simulink model "HelicPlantMRAC"  (R2023b)
settings: Solver=ode45  StartTime=0.0  StopTime=100  RelTol=1e-3  EnableMultiTasking=on
values from neighbouring files (symbols this model uses):
  am = -4.0    (= -4)    [int.m]
  bbar = -1    [int.m]
  bm = 4.0    (= 4)    [int.m]
  gammaphi = 0.1    [int.m]
  gammar = 0.0005    [int.m]
  gammax = 0.0005    [int.m]
  ke = 10    [int.m]
  khat0 = 0    [int.m]
  lhat0 = 0    [int.m]
  p = -1/(2*am)    (= 0.125)    [int.m]
  R = 0.15    [int.m]
  sigma2e = 0.0    (= 0)    [int.m]
  Tc = 0.1    [int.m]
  thetahat0 = 0    [int.m]
  wr = 0.25    [int.m]
libraries: simulink x1
settings Model: Creator=Abel  LastModifiedBy=Abel
settings SolverCC: AlgebraicLoopSolver=TrustRegion
settings DataIOCC: LimitDataPoints=on  SaveFormat=Array  SignalLoggingSaveFormat=ModelDataLogs  ReturnWorkspaceOutputs=off
settings OptimizationCC: InitFltsAndDblsToZero=on  LifeSpan=inf
settings DebuggingCC: SaveWithParameterizedLinksMsg=none  UnderspecifiedInitializationDetection=Classic  MergeDetectMultiDrivingBlocksExec=none  SignalResolutionControl=TryResolveAllWithWarning  SolverPrmCheckMsg=warning  MultiTaskDSMMsg=warning  MultiTaskCondExecSysMsg=none  FcnCallInpInsideContextMsg=warning  UnconnectedInputMsg=warning  UnconnectedOutputMsg=warning  UnconnectedLineMsg=warning  SFUnexpectedBacktrackingDiag=warning  SFNoUnconditionalDefaultTransitionDiag=warning  SFExecutionAtInitializationDiag=none  ArithmeticOperatorsInVariantConditions=warning
settings HardwareCC: ProdBitPerPointer=32  ProdBitPerSizeT=32  ProdBitPerPtrDiffT=32  ProdLargestAtomicFloat=None  ProdIntDivRoundTo=Undefined  ProdEndianess=Unspecified  ProdWordSize=32  ProdHWDeviceType=32-bit Generic
settings ModelReferenceCC: PropagateSignalLabelsOutOfModel=off
settings CodeAppCC: StateflowObjectComments=on
settings GRTTargetCC: TargetFcnLib=ansi_tfl_tmw.mat  TargetLangStandard=C89/C90 (ANSI)  CombineOutputUpdateFcns=off  GRTInterface=on
settings ConfigComp: CovMetricSettings=dw  CovSaveCumulativeToWorkspaceVar=on  CovSaveSingleToWorkspaceVar=on

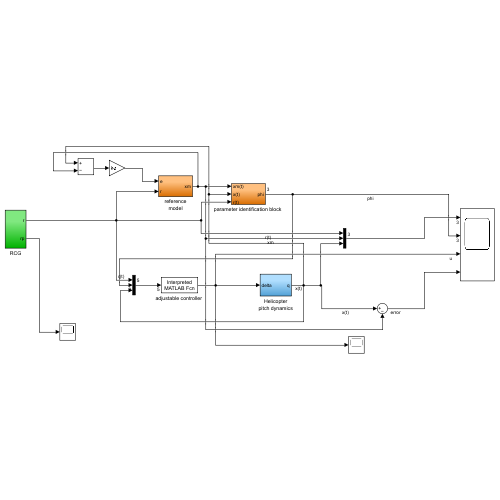
[thumbnail: Simulink's stored preview of the top-level diagram]
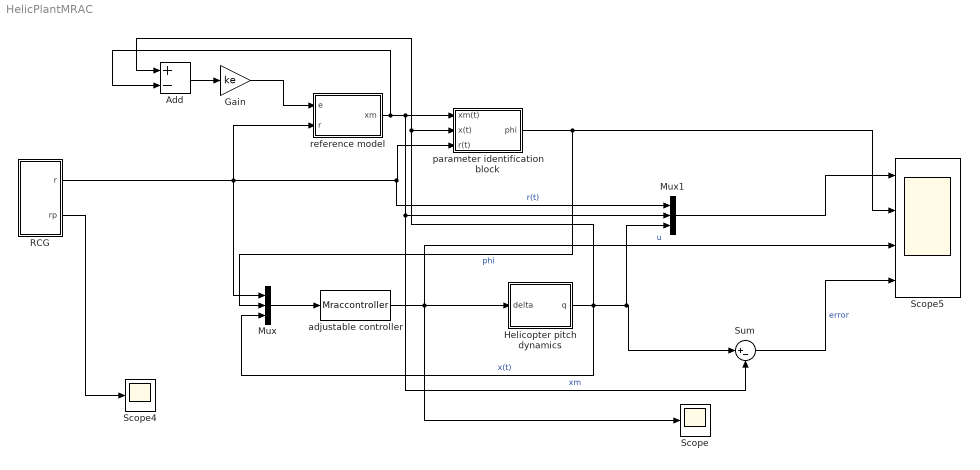
== system HelicPlantMRAC ==
  Add : Sum  Inputs=+-
  Gain : Gain  Gain=ke
  Helicopter pitch dynamics : Subsystem
  Mux : Mux  Inputs=[1 3 1]
  Mux1 : Mux  Inputs=3
  RCG : Subsystem
  Scope : Scope
  Scope4 : Scope
  Scope5 : Scope  NumInputPorts=4
  Sum : Sum  Inputs=|+-
  "adjustable controller " : MATLABFcn  MATLABFcn=Mraccontroller  OutputDimensions=1
  "parameter identification block " : Subsystem
  reference model : Subsystem
  wires:
  RCG/1(r) -> Mux/1, Mux1/1, "parameter identification block "/3(r(t)), reference model/2(r)  "r(t)"
  reference model/1(xm) -> Add/2, Sum/2, Mux1/2, "parameter identification block "/1(xm(t))  "xm"
  Helicopter pitch dynamics/1(q) -> Mux1/3, Sum/1, Mux/3, Add/1, "parameter identification block "/2(x(t))  "x(t)"
  "adjustable controller "/1 -> Scope5/3, Helicopter pitch dynamics/1(delta), Scope/1  "u"
  "parameter identification block "/1(phi) -> Scope5/2, Mux/2  "phi"
  Mux/1 -> "adjustable controller "/1
  RCG/2(rp) -> Scope4/1
  Add/1 -> Gain/1
  Gain/1 -> reference model/1(e)
  Mux1/1 -> Scope5/1
  Sum/1 -> Scope5/4  "error"

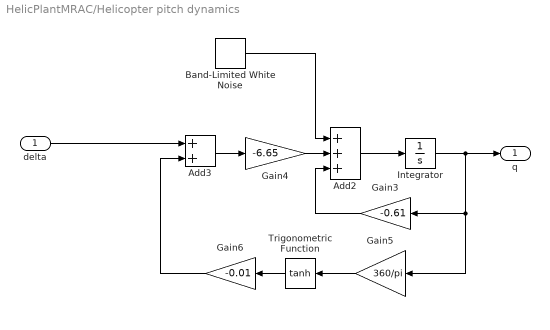
== system HelicPlantMRAC/Helicopter pitch dynamics ==
  delta : Inport
  Add2 : Sum  Inputs=+++
  Add3 : Sum
  Band-Limited White Noise : simulink/Sources/Band-Limited White Noise  Cov=[sigma2e*Tc]  Ts=Tc  seed=[23341]
  Gain3 : Gain  Gain=-0.61
  Gain4 : Gain  Gain=-6.65
  Gain5 : Gain  Gain=360/pi
  Gain6 : Gain  Gain=-0.01
  Integrator : Integrator
  Trigonometric Function : Trigonometry  Operator=tanh
  q : Outport
  wires:
  Integrator/1 -> Gain3/1, Gain5/1, q/1
  Add2/1 -> Integrator/1
  Gain5/1 -> Trigonometric Function/1
  Trigonometric Function/1 -> Gain6/1
  Add3/1 -> Gain4/1
  Gain6/1 -> Add3/2
  delta/1 -> Add3/1
  Gain3/1 -> Add2/3
  Gain4/1 -> Add2/2
  Band-Limited White Noise/1 -> Add2/1

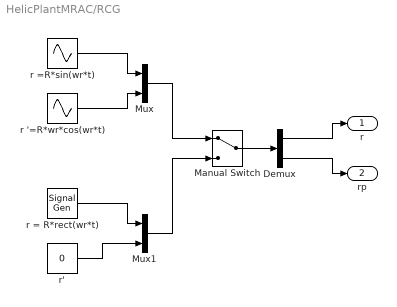
== system HelicPlantMRAC/RCG ==
  Demux : Demux  Outputs=2
  Manual Switch : ManualSwitch
  Mux : Mux  Inputs=2
  Mux1 : Mux  Inputs=2
  r '=R*wr*cos(wr*t) : Sin  Amplitude=R*wr  Frequency=wr  Phase=pi/2  SampleTime=Tc
  r = R*rect(wr*t) : SignalGenerator  WaveForm=square  Amplitude=R  Frequency=wr  Units=rad/sec
  r =R*sin(wr*t) : Sin  Amplitude=R  Frequency=wr  SampleTime=Tc
  r' : Constant  Value=0
  r : Outport
  rp : Outport  Port=2
  wires:
  r =R*sin(wr*t)/1 -> Mux/1
  r '=R*wr*cos(wr*t)/1 -> Mux/2
  r = R*rect(wr*t)/1 -> Mux1/1
  r'/1 -> Mux1/2
  Mux/1 -> Manual Switch/1
  Mux1/1 -> Manual Switch/2
  Manual Switch/1 -> Demux/1
  Demux/1 -> r/1
  Demux/2 -> rp/1

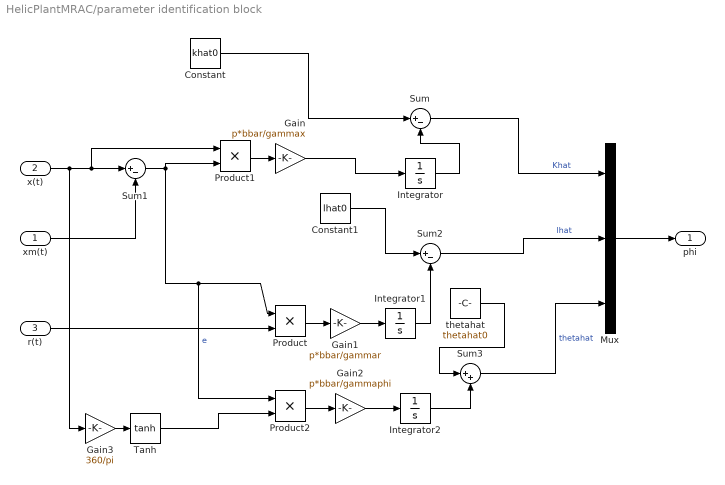
== system HelicPlantMRAC/parameter identification block  ==
  xm(t) : Inport
  x(t) : Inport  Port=2
  r(t) : Inport  Port=3
  Constant : Constant  Value=khat0
  Constant1 : Constant  Value=lhat0
  Gain : Gain  Gain=p*bbar/gammax
  Gain1 : Gain  Gain=p*bbar/gammar
  Gain2 : Gain  Gain=p*bbar/gammaphi
  Gain3 : Gain  Gain=360/pi
  Integrator : Integrator
  Integrator1 : Integrator
  Integrator2 : Integrator
  Mux : Mux  Inputs=3
  Product : Product
  Product1 : Product
  Product2 : Product
  Sum : Sum  Inputs=|+-
  Sum1 : Sum  Inputs=|+-
  Sum2 : Sum  Inputs=|+-
  Sum3 : Sum  Inputs=|++
  Tanh : Trigonometry  Operator=tanh
  thetahat : Constant  Value=thetahat0
  phi : Outport
  wires:
  Constant/1 -> Sum/1
  x(t)/1 -> Gain3/1, Product1/1, Sum1/1
  xm(t)/1 -> Sum1/2
  Sum1/1 -> Product2/1, Product/1, Product1/2  "e"
  Integrator/1 -> Sum/2
  Sum/1 -> Mux/1  "Khat"
  Constant1/1 -> Sum2/1
  Integrator1/1 -> Sum2/2
  Sum2/1 -> Mux/2  "lhat"
  thetahat/1 -> Sum3/1
  Sum3/1 -> Mux/3  "thetahat"
  Gain3/1 -> Tanh/1
  Integrator2/1 -> Sum3/2
  Mux/1 -> phi/1
  Product1/1 -> Gain/1
  Gain/1 -> Integrator/1
  Product/1 -> Gain1/1
  Gain1/1 -> Integrator1/1
  r(t)/1 -> Product/2
  Product2/1 -> Gain2/1
  Gain2/1 -> Integrator2/1
  Tanh/1 -> Product2/2

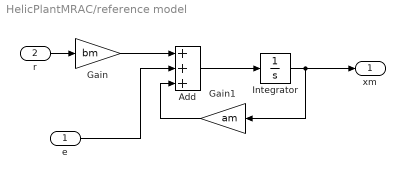
== system HelicPlantMRAC/reference model ==
  e : Inport
  r : Inport  Port=2
  Add : Sum  Inputs=+++
  Gain : Gain  Gain=bm
  Gain1 : Gain  Gain=am
  Integrator : Integrator
  xm : Outport
  wires:
  Gain/1 -> Add/1
  Add/1 -> Integrator/1
  Integrator/1 -> Gain1/1, xm/1
  r/1 -> Gain/1
  Gain1/1 -> Add/3
  e/1 -> Add/2
